simulink model "PMW_SPWM"  (R2025b)
settings: Solver=VariableStepAuto  StartTime=0.0  StopTime=10.0  RelTol=1e-3
libraries: simulink x1
settings Model: Creator=night  LastModifiedBy=night

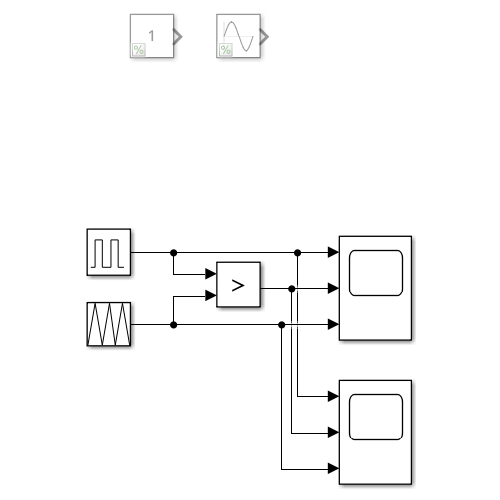
[thumbnail: Simulink's stored preview of the top-level diagram]
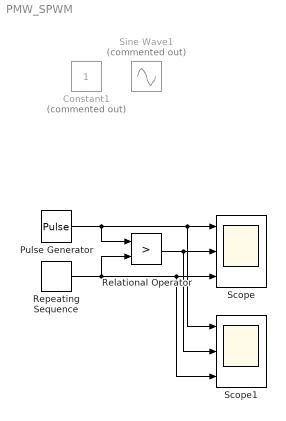
== system PMW_SPWM ==
  Constant1 : Constant  Commented=on
  Pulse Generator : DiscretePulseGenerator  PulseType=Time based  Period=5  PulseWidth=20
  Relational Operator : RelationalOperator  Operator=>  OutDataTypeStr=boolean  RndMeth=Simplest  InputSameDT=off
  Repeating Sequence : simulink/Sources/Repeating Sequence  rep_seq_t=[0 0.5 1]  rep_seq_y=[0 2 0]
  Scope : Scope  NumInputPorts=3
      settings: ActiveDisplayYMinimum=0.9  ActiveDisplayYMaximum=1.1
  Scope1 : Scope  NumInputPorts=3
      settings: ActiveDisplayYMinimum=-0.24999999999999994  ActiveDisplayYMaximum=2.25
  Sine Wave1 : Sin  Commented=on  SampleTime=0
  wires:
  Pulse Generator/1 -> Scope1/1, Scope/1, Relational Operator/1
  Repeating Sequence/1 -> Relational Operator/2, Scope1/3, Scope/3
  Relational Operator/1 -> Scope1/2, Scope/2
